simulink model "vvv"  (Simulink 7.9)
settings: Solver=ode45  StartTime=0.0  StopTime=20  RelTol=1e-3
libraries: dspsrcs4 x2, commsink2 x1, commfilt2 x1, commdigbbndam3 x1, commtimrec2 x1
settings Model: Creator=Estilo  LastModifiedBy=Estilo

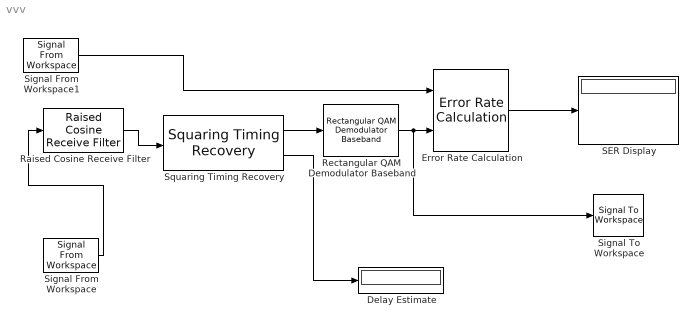
== system vvv ==
  Delay Estimate : Display
  Error Rate Calculation : commsink2/Error Rate Calculation  N=2*4  st_delay=0  cp_mode=Entire frame  subframe=[]  PMode=Port  WsName=ErrorVec  RsMode2=off  stop=off  numErr=100  maxBits=1e6
  Raised Cosine Receive Filter : commfilt2/Raised Cosine Receive Filter  filtType=Square root  N=8  D=4  R=0.2  sampMode=Mute  saveAsFlag=0  rateMode=None  downFactor=8  downOffset=0  framing=Maintain input frame rate  InputProcessing=Columns as channels (frame based)  checkGain=Normalized  filterGain=1  checkCoeff=off  variableName=rcRxFilt  launchFVT=off  roundingMode=Floor  overflowMode=off
  Rectangular QAM Demodulator Baseband : commdigbbndam3/Rectangular QAM Demodulator Baseband  M=16  PowType=Peak Power  MinDist=2  AvgPow=1  PeakPow=1  Ph=0  Dec=Binary  Mapping=[0:15]  OutType=Integer  DecType=Hard decision  VarSource=Dialog  Variance=1  outDtype1=double  outDtype2=double  derotateFactorWordLen=16  denormFactorWordLen=16  prodOutWordLen=32  prodOutRoundingMode=Floor  prodOutOverflowMode=Wrap  sumWordLen=32
  SER Display : Display
  Signal From Workspace : dspsrcs4/Signal From Workspace  X=yout  Ts=1/1000  nsamps=800  OutputAfterFinalValue=Setting to zero  ignoreOrWarnInputAndFrameLengths=off
  Signal From Workspace1 : dspsrcs4/Signal From Workspace  X=yout1  Ts=1/1000  nsamps=100  OutputAfterFinalValue=Setting to zero  ignoreOrWarnInputAndFrameLengths=off
  Signal To Workspace : SignalToWorkspace  VariableName=yout3
      settings: CopyFcn=dspblkcopystw(gcbh);
  Squaring Timing Recovery : commtimrec2/Squaring Timing Recovery  numSymb=100  sampPerSymb=8
  wires:
  Signal From Workspace/1 -> Raised Cosine Receive Filter/1
  Raised Cosine Receive Filter/1 -> Squaring Timing Recovery/1
  Squaring Timing Recovery/2 -> Delay Estimate/1
  Signal From Workspace1/1 -> Error Rate Calculation/1
  Squaring Timing Recovery/1 -> Rectangular QAM Demodulator Baseband/1
  Rectangular QAM Demodulator Baseband/1 -> Error Rate Calculation/2, Signal To Workspace/1
  Error Rate Calculation/1 -> SER Display/1
